simulink model "DCmotor0904"  (R2022a)
settings: Solver=VariableStepAuto  StartTime=0.0  StopTime=1  MaxStep=1e-6  RelTol=1e-3
values from neighbouring files (symbols this model uses):
  IaN = TN / Ct_phi    (= 103.333333333)    [DC_PWM.m]
  Ki_cur = Ki / ti    (= 750)    [DC_PWM.m]
  Ki_spd = Kn / tn    (= 112.225389146)    [DC_PWM.m]
  Kp_cur = Ki    (= 15)    [DC_PWM.m]
  Kp_spd = Kn    (= 0.808022801849)    [DC_PWM.m]
  nN = 0.8*n0    (= 1315.68086289)    [DC_PWM.m]
  TA = 4*Tsumn + Tfn    (= 0.0082)    [DC_PWM.m]
  TB = Tfi    (= 0.0002)    [DC_PWM.m]
  Tfi = 200e-6    (= 0.0002)    [DC_PWM.m]
  Tfn = 1e-3    (= 0.001)    [DC_PWM.m]
  TN = ((Udc-nN*Ce_phi)*Ct_phi)/Ra    (= 186)    [DC_PWM.m]
  Udc = 310    [DC_PWM.m]
libraries: spsIGBTDiodeLib x4, spsGroundLib x3, spsDCVoltageSourceLib x2, spsDCMachineLib x1, simulink x1, spsVoltageMeasurementLib x1, spspowerguiLib x1
settings Model: Creator=DELL  LastModifiedBy=57308
settings SolverCC: AlgebraicLoopSolver=TrustRegion
settings DataIOCC: ReturnWorkspaceOutputs=off
settings DebuggingCC: UnconnectedInputMsg=warning  UnconnectedOutputMsg=warning  UnconnectedLineMsg=warning  SFMachineParentedDataDiag=warning  ArithmeticOperatorsInVariantConditions=warning
settings SFSimCC: SimUseLocalCustomCode=off  CustomCodeUndefinedFunction=UseInterfaceOnly
settings RTWCC: RTWUseLocalCustomCode=off
settings CodeAppCC: StateflowObjectComments=on
settings SimscapeCC: SimscapeNormalizeSystem=off

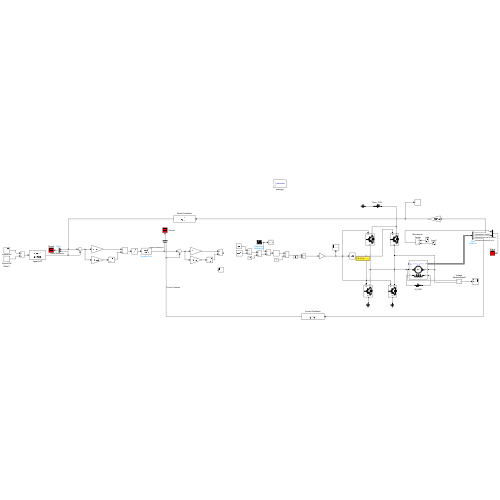
[thumbnail: Simulink's stored preview of the top-level diagram]
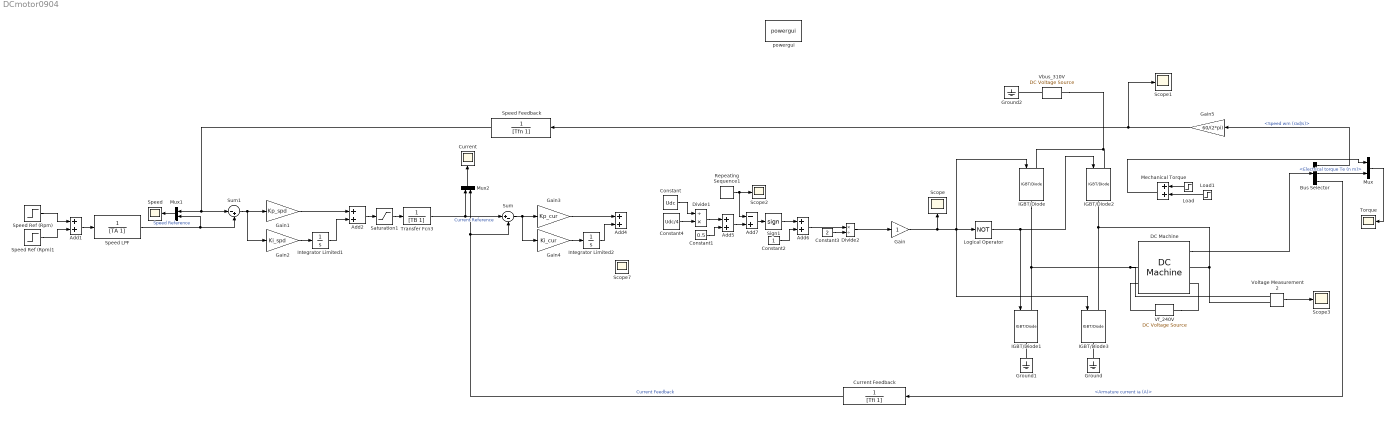
== system DCmotor0904 ==
  Add{1..2,4..6} (5 alike) : Sum
  Add7 : Sum  Inputs=-+
  Bus Selector : BusSelector  OutputSignals=Speed wm (rad/s),Electrical torque Te (n m),Armature current ia (A)
  Constant : Constant  Value=Udc
  Constant1 : Constant  Value=0.5
  Constant2 : Constant
  Constant3 : Constant  Value=2
  Constant4 : Constant  Value=Udc/4
  Current : Scope
  Current Feedback : TransferFcn  Denominator=[Tfi 1]
  DC Machine : spsDCMachineLib/DC Machine  PresetModel=No  MechanicalLoad=Torque TL  FieldType=Wound  ShowDetailedParameters=on  MeasurementBus=off  RLa="[ 0.6  0.012]"  RLf="[ 240  120]"  Laf=1.8  MachineConstant=Torque constant (N.m/A)  Ke=1.8  Kt=1.8  J=0.05  Bm=0  Tf=0  w0=1  Ifinit=1  TsPowergui=0  TsBlock=-1
  Divide1 : Product  Inputs=/*
  Divide2 : Product  Inputs=*/
  Gain : Gain
  Gain1 : Gain  Gain=Kp_spd
  Gain2 : Gain  Gain=Ki_spd
  Gain3 : Gain  Gain=Kp_cur
  Gain4 : Gain  Gain=Ki_cur
  Gain5 : Gain  Gain=60/(2*pi)
  Ground : spsGroundLib/Ground  LConnTagsString=a
  Ground1 : spsGroundLib/Ground  LConnTagsString=a
  Ground2 : spsGroundLib/Ground  LConnTagsString=a
  IGBT/Diode{,1..3} (4 alike) : spsIGBTDiodeLib/IGBT//Diode  Ron=1e-3  Rs=1e5  Cs=inf  Measurements=off
  Integrator Limited1 : Integrator  LimitOutput=on  UpperSaturationLimit=2*IaN  LowerSaturationLimit=0
  Integrator Limited2 : Integrator  LimitOutput=on  UpperSaturationLimit=2*IaN  LowerSaturationLimit=0
  Load : Step  Time=0.4  After=TN  SampleTime=0
  Load1 : Step  Time=0.6  After=-0.2*TN  SampleTime=0
  Logical Operator : Logic  Operator=NOT  AllPortsSameDT=off  OutDataTypeStr=boolean
  Mechanical Torque : Sum
  Mux : Mux  Inputs=2
  Mux1 : Mux  Inputs=2
  Mux2 : Mux  Inputs=2
  Repeating Sequence1 : simulink/Sources/Repeating Sequence  rep_seq_t=[0 100e-6 200e-6]  rep_seq_y=[0 1 0]
  Saturation1 : Saturate  UpperLimit=2*IaN  LowerLimit=-2*IaN
  Scope{,1..3,7} (5 alike) : Scope
  Sign1 : Signum
  Speed : Scope
  Speed Feedback : TransferFcn  Denominator=[Tfn 1]
  Speed LPF : TransferFcn  Denominator=[TA 1]
  Speed Ref (Rpm) : Step  Time=0.2  After=0.8*nN  SampleTime=0
  Speed Ref (Rpm)1 : Step  Time=0.8  After=-0.3*nN  SampleTime=0  VectorParams1D=off
  Sum : Sum  Inputs=|+-
  Sum1 : Sum  Inputs=|-+
  Torque : Scope
  Transfer Fcn3 : TransferFcn  Denominator=[TB 1]
  Vbus_310V : spsDCVoltageSourceLib/DC Voltage Source  Amplitude=Udc  Measurements=None
  Vf_240V : spsDCVoltageSourceLib/DC Voltage Source  Amplitude=240  Measurements=None
  Voltage Measurement2 : spsVoltageMeasurementLib/Voltage Measurement  PhasorSimulation=off  OutputType=Complex  PSBequivalent=0
  powergui : spspowerguiLib/powergui  Priority=1  SimulationMode=Continuous  SampleTime=50e-6  frequency=60  Iterations=50  frequencyindice=0  Pbase=100e6  ErrMax=1e-4  UnitsV=kV  UnitsW=MW  buscounter=0  FunctionMessages=off  echomessages=off  EnableUseOfTLC=off  CurrentSourceSwitches=on  DisableSnubberDevices=off  DisableRonSwitches=off  DisableVfSwitches=off  DisplayEquations=off  AutomaticDiscreteSolvers=off  SolverType=Tustin/Backward Euler (TBE)  Interpol=off  ExternalGateDelay=off  methode=off  Ts=10  x0status=blocks  SPID=off  SwTol=0  HookPort=off  NonlinearTolerance=1e-4  nMaxIteration=100  ContinueOnMaxIteration=off  RestoreLinks=warning  ResistiveCurrentMeasurement=off  Frange=[0:2:500]  Ylog=off  Xlog=on  ShowGrid=off  save=off  variable=ZData  structure=0  ZoomFFT=off  StartTime=0.0  cycles=1  DisplayStyle=1  fundamental=60  FreqAxis=off  MaxFrequency=1000  frequencyindicesteady=1  RmsSteady=1  display=off
  wires:
  Gain2/1 -> Integrator Limited1/1
  Sum1/1 -> Gain2/1, Gain1/1
  Integrator Limited1/1 -> Add2/2
  Add2/1 -> Saturation1/1
  Saturation1/1 -> Transfer Fcn3/1
  Gain1/1 -> Add2/1
  Transfer Fcn3/1 -> Mux2/1, Sum/1  "Current Reference"
  Sum/1 -> Gain4/1, Gain3/1
  Gain4/1 -> Integrator Limited2/1
  Gain3/1 -> Add4/1
  Integrator Limited2/1 -> Add4/2
  Divide1/1 -> Add5/1
  Constant1/1 -> Add5/2
  Sign1/1 -> Add6/1
  Constant2/1 -> Add6/2
  Add5/1 -> Add7/2
  Repeating Sequence1/1 -> Scope2/1, Add7/1
  Add6/1 -> Divide2/1
  Constant3/1 -> Divide2/2
  Add7/1 -> Sign1/1
  DC Machine/1 -> Bus Selector/1
  Bus Selector/1 -> Gain5/1  "<Speed wm (rad/s)>"
  Bus Selector/2 -> Mux/2  "<Electrical torque Te (n m)>"
  Gain5/1 -> Scope1/1, Speed Feedback/1
  Speed LPF/1 -> Sum1/2, Mux1/2  "Speed Reference"
  Speed Feedback/1 -> Mux1/1, Sum1/1
  Current Feedback/1 -> Mux2/2, Sum/2  "Current Feedback"
  Mux1/1 -> Speed/1
  Mux2/1 -> Current/1
  Mux/1 -> Torque/1
  Add1/1 -> Speed LPF/1
  Speed Ref (Rpm)/1 -> Add1/1
  Speed Ref (Rpm)1/1 -> Add1/2
  Mechanical Torque/1 -> Mux/1
  Load/1 -> Mechanical Torque/1
  Load1/1 -> Mechanical Torque/2
  Gain/1 -> IGBT/Diode/1, Logical Operator/1, IGBT/Diode3/1, Scope/1
  Voltage Measurement2/1 -> Scope3/1
  Divide2/1 -> Gain/1
  Bus Selector/3 -> Current Feedback/1  "<Armature current ia (A)>"
  Logical Operator/1 -> IGBT/Diode1/1, IGBT/Diode2/1
  Constant/1 -> Divide1/1
  Constant4/1 -> Divide1/2
  connections:
  IGBT/Diode/RConn1 -- Voltage Measurement2/LConn1 -- DC Machine/LConn1 -- IGBT/Diode1/LConn1
  Vf_240V/RConn1 -- DC Machine/LConn2
  Vf_240V/LConn1 -- DC Machine/RConn2
  IGBT/Diode3/LConn1 -- IGBT/Diode2/RConn1 -- Voltage Measurement2/LConn2 -- DC Machine/RConn1
  IGBT/Diode2/LConn1 -- IGBT/Diode/LConn1 -- Vbus_310V/RConn1
  Vbus_310V/LConn1 -- Ground2/LConn1
  Ground1/LConn1 -- IGBT/Diode1/RConn1
  Ground/LConn1 -- IGBT/Diode3/RConn1
